simulink model "Testzisxplusy"  (R2017b)
settings: Solver=FixedStepAuto  StartTime=0.0  StopTime=10.0  FixedStep=1  RelTol=1e-3
settings Model: Creator=georgimarkov  LastModifiedBy=georgimarkov

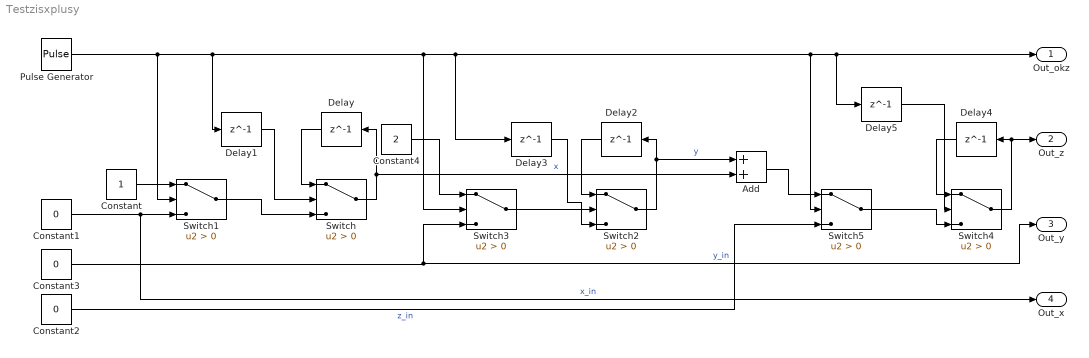
== system Testzisxplusy ==
  Add : Sum
  Constant : Constant
  Constant1 : Constant  Value=0
  Constant2 : Constant  Value=0
  Constant3 : Constant  Value=0
  Constant4 : Constant  Value=2
  Delay{,1..5} (6 alike) : Delay  DelayLength=1  InitialCondition=0
  Pulse Generator : DiscretePulseGenerator  PulseType=Time based  Period=10  PulseWidth=10  PhaseDelay=1
  Switch{,1..5} (6 alike) : Switch  Criteria=u2 > Threshold
  Out_okz : Outport
  Out_z : Outport  Port=2
  Out_y : Outport  Port=3
  Out_x : Outport  Port=4
  wires:
  Delay/1 -> Switch/1
  Delay1/1 -> Switch/2
  Constant1/1 -> Out_x/1, Switch1/3  "x_in"
  Constant/1 -> Switch1/1
  Switch1/1 -> Switch/3
  Switch/1 -> Add/2, Delay/1  "x"
  Pulse Generator/1 -> Switch1/2, Delay1/1, Switch3/2, Switch5/2, Delay5/1, Out_okz/1, Delay3/1
  Switch2/1 -> Delay2/1, Add/1  "y"
  Constant3/1 -> Out_y/1, Switch3/3  "y_in"
  Delay2/1 -> Switch2/1
  Delay3/1 -> Switch2/2
  Switch3/1 -> Switch2/3
  Switch5/1 -> Switch4/3
  Delay5/1 -> Switch4/2
  Delay4/1 -> Switch4/1
  Switch4/1 -> Out_z/1, Delay4/1
  Add/1 -> Switch5/1
  Constant2/1 -> Switch5/3  "z_in"
  Constant4/1 -> Switch3/1
